simulink model "work5"  (R2026a)
settings: Solver=ode45  StopTime=10  RelTol=1e-6  AbsTol=1e-8
undefined symbols (not defined in the file or in its folder): A_obs, B_obs, cholW, minusK
libraries: simulink x2
settings Model: Creator=m  LastModifiedBy=m

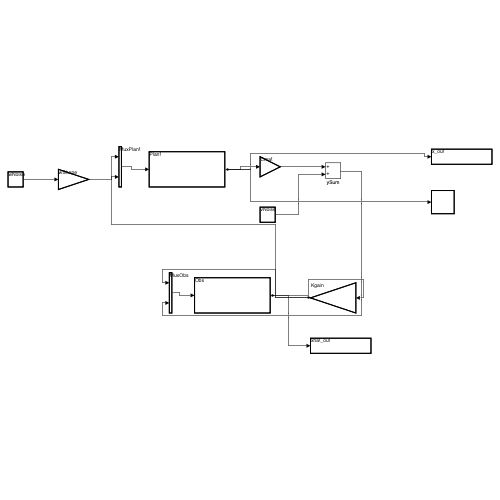
[thumbnail: Simulink's stored preview of the top-level diagram]
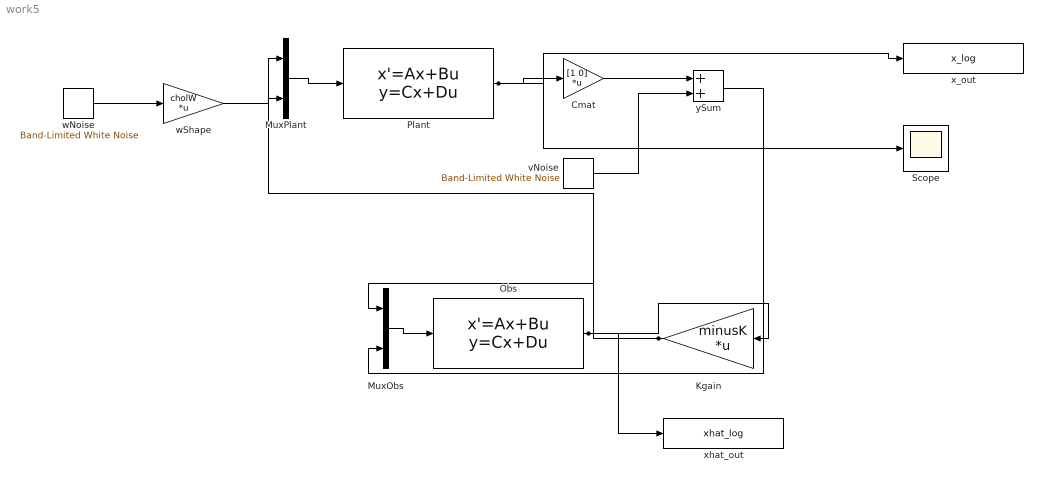
== system work5 ==
  Cmat : Gain  Gain=[1 0]  Multiplication=Matrix(K*u)
  Kgain : Gain  Gain=minusK  Multiplication=Matrix(K*u)
  MuxObs : Mux  Inputs=2
  MuxPlant : Mux  Inputs=2
  Obs : StateSpace  A=A_obs  B=B_obs  C=[1 0;0 1]  D=[0 0;0 0]  InitialCondition=[0;0]
  Plant : StateSpace  A=[0 -4;1 -4]  B=[8 1 0;7 0 1]  C=[1 0;0 1]  D=[0 0 0;0 0 0]  InitialCondition=[1;0]
  Scope : Scope
  vNoise : simulink/Sources/Band-Limited White Noise  Cov=5  Ts=0.01  seed=99001
  wNoise : simulink/Sources/Band-Limited White Noise  Cov=[1 1]  Ts=0.01  seed=[23341 23342]
  wShape : Gain  Gain=cholW  Multiplication=Matrix(K*u)
  x_out : ToWorkspace  VariableName=x_log  SaveFormat=Timeseries  SampleTime=-1
  xhat_out : ToWorkspace  VariableName=xhat_log  SaveFormat=Timeseries  SampleTime=-1
  ySum : Sum
  wires:
  Kgain/1 -> MuxPlant/1, MuxObs/1
  wShape/1 -> MuxPlant/2
  wNoise/1 -> wShape/1
  MuxPlant/1 -> Plant/1
  Plant/1 -> Cmat/1, x_out/1, Scope/1
  Cmat/1 -> ySum/1
  vNoise/1 -> ySum/2
  ySum/1 -> MuxObs/2
  MuxObs/1 -> Obs/1
  Obs/1 -> Kgain/1, xhat_out/1
